simulink model "ARC_DTm"  (R2025b)
settings: Solver=FixedStepAuto  StartTime=0.0  StopTime=10080  FixedStep=1  RelTol=1e-3
PreLoadFcn:
  | %For Preload, set the working path
  | modelFolder = fileparts(which(bdroot));
  | addpath(genpath(modelFolder));
StartFcn:
  | tic
StopFcn:
  | fprintf("Sim Time: %.02f min", toc/60)
values from neighbouring files (symbols this model uses):
  batteryScenario = p.batteryScenario    [RUNSIM_ParameterSweep.m]    (also in _RUNSIM_ParameterSweep.m)
  Electricity_SalePriceModifier = 50/100    (= 0.5)    [RUNSIM_ParameterSweep.m]    (also in _RUNSIM_ParameterSweep.m)
  LUT = LUT_load.gamLUT    [RUNSIM_ParameterSweep.m]    (also in _RUNSIM_ParameterSweep.m)
  minimum_UF_system_flow = 5833    [RUNSIM_ParameterSweep.m]    (also in _RUNSIM_ParameterSweep.m)
  PROS1_recoveryrate = 61    [RUNSIM_ParameterSweep.m]    (also in _RUNSIM_ParameterSweep.m)
  PROS2_recoveryrate = 62    [RUNSIM_ParameterSweep.m]    (also in _RUNSIM_ParameterSweep.m)
  ROstabilization_time = p.ROstabilization_time    [RUNSIM_ParameterSweep.m]    (also in _RUNSIM_ParameterSweep.m)
  solarModifier = maximum_solar_generation / 300    [RUNSIM_ParameterSweep.m]    (also in _RUNSIM_ParameterSweep.m)
  TSRO_recoveryrate = 51    [RUNSIM_ParameterSweep.m]    (also in _RUNSIM_ParameterSweep.m)
  UF_RecoveryRate = 96    [RUNSIM_ParameterSweep.m]    (also in _RUNSIM_ParameterSweep.m)
undefined symbols (not defined in the file or in its folder): A_PROS1, A_PROS2, A_TSRO, B_PROS1, B_PROS2, B_TSRO, BW_Max_Time, BW_Max_Vol_gal, CEB_Max_Time, CEB_Max_Vol_gal, CIP_Max_Time, E, FF, h, L, w
libraries: simulink x40
(part 1 of 11)
settings Model: Creator=joshl  LastModifiedBy=joshl
settings DebuggingCC: AlgebraicLoopMsg=none  IntegerOverflowMsg=none
settings RTWCC: GenCodeOnly=on

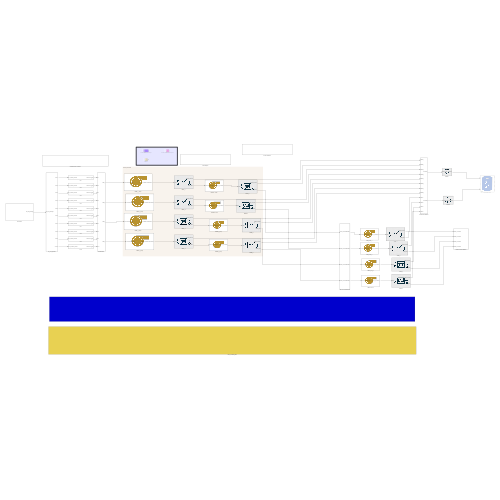
[thumbnail: Simulink's stored preview of the top-level diagram]
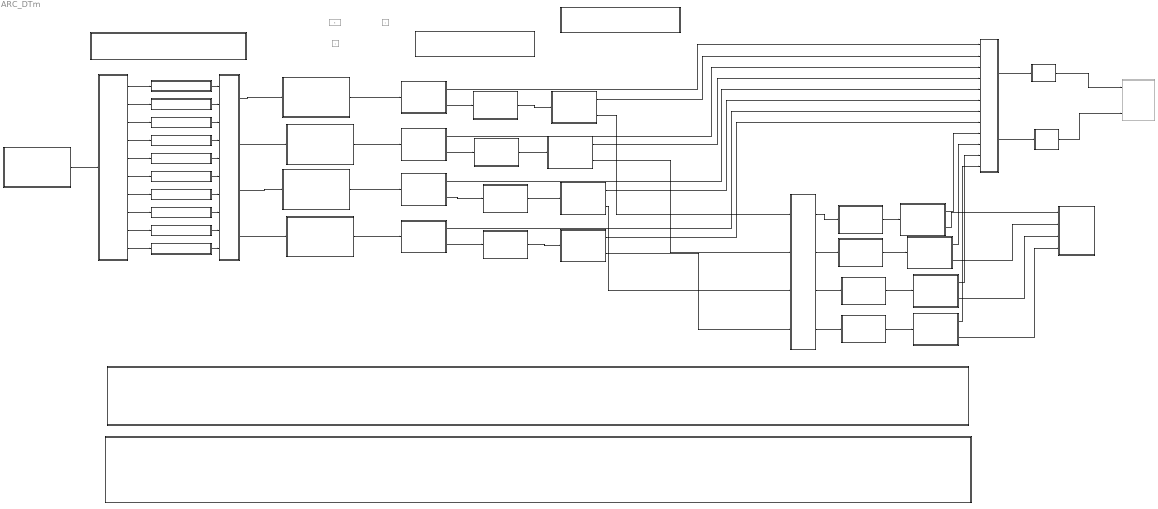
== system ARC_DTm ==
  note: Primary RO Skids
  note: LEGEND
  Constant Value from Analysis : Constant  Commented=on  Value=E
  Constant Value from Plant Specs : Constant  Commented=on
  PRO Concentrate Manifold : Subsystem
  PRO Manifolds : Subsystem
  PROS1_1 : Subsystem
      mask Display: image('ROmodule.png');
  PROS1_1_Pump : Subsystem
      mask Display: image('HydraulicPump.png');
  PROS1_2 : Subsystem
      mask Display: image('ROmodule.png');
  PROS1_2_Pump : Subsystem
      mask Display: image('HydraulicPump.png');
  PROS1_3 : Subsystem
      mask Display: image('ROmodule.png');
  PROS1_3_Pump : Subsystem
      mask Display: image('HydraulicPump.png');
  PROS1_4 : Subsystem
      mask Display: image('ROmodule.png');
  PROS1_4_Pump : Subsystem
      mask Display: image('HydraulicPump.png');
  PROS2_1 : Subsystem
      mask Display: image('ROmodule.png');
  PROS2_1_Pump : Subsystem
      mask Display: image('HydraulicPump.png');
  PROS2_2 : Subsystem
      mask Display: image('ROmodule.png');
  PROS2_2_Pump : Subsystem
      mask Display: image('HydraulicPump.png');
  PROS2_3 : Subsystem
      mask Display: image('ROmodule.png');
  PROS2_3_Pump : Subsystem
      mask Display: image('HydraulicPump.png');
  PROS2_4 : Subsystem
      mask Display: image('ROmodule.png');
  PROS2_4_Pump : Subsystem
      mask Display: image('HydraulicPump.png');
  Plant Setpoints : Subsystem
  Plant_LocalLoad_FMU : Subsystem
  Process Constants : Subsystem
  Product Water Tank : Subsystem  Commented=on  mask{lid=Closed, area=100, vol=500, volMax=0.750, volMin=.25, initVol=0.720, initTSS=43.0, InitSal=24.500, initT=31.500}
      mask prompts: lid "Open or Closed Lid?"; area "Surface Area of Tank (ft^2)"; vol "Volume of Tank (gal)"; volMax "Operational Max Volume (%)"; volMin "Operational Min Volume (%)"; initVol "Initial Storage Volume (%)"; initTSS "Initial TSS (ppm)"; InitSal "Initial Salinity (ppm)"; initT "Initial Temperature (*C)"
      mask TypeOptions lid: Open | Closed
      mask DialogControl Control1 Prompt: Raw Water Tank geometry definition
      mask Display: image('C:\Users\joshl\OneDrive - Colostate\Research\NAWI\Simulink Model\Icons\RawWaterTank.png'); % Use "Edit Image" on toolstrip to change.
  RO Permeate Manifold : Subsystem
  Setpoint : Constant  Commented=on
  Subsystem1 : Subsystem
  TSRO Concentrate Manifold : Subsystem
  TSRO_1 : Subsystem
      mask Display: image('ROmodule.png');
  TSRO_2 : Subsystem
      mask Display: image('ROmodule.png');
  TSRO_3 : Subsystem
      mask Display: image('ROmodule.png');
  TSRO_4 : Subsystem
      mask Display: image('ROmodule.png');
  TSRO_Pump_1 : Subsystem
      mask Display: image('HydraulicPump.png');
  TSRO_Pump_2 : Subsystem
      mask Display: image('HydraulicPump.png');
  TSRO_Pump_3 : Subsystem
      mask Display: image('HydraulicPump.png');
  TSRO_Pump_4 : Subsystem
      mask Display: image('HydraulicPump.png');
  UF Maintenance Coordinator : Subsystem
  UF Pumping : Subsystem
  UF1 : Subsystem
  UF10 : Subsystem
  UF2 : Subsystem
  UF3 : Subsystem
  UF4 : Subsystem
  UF5 : Subsystem
  UF6 : Subsystem
  UF7 : Subsystem
  UF8 : Subsystem
  UF9 : Subsystem
  UF_Feed_Manifold : Subsystem
  UVAOP 1 : Subsystem
      mask Display: image('11bcd1e1-7ab0-44c4-a430-d02249a16220.png');
  UVAOP 2 : Subsystem
      mask Display: image('11bcd1e1-7ab0-44c4-a430-d02249a16220.png');
  wires:
  PROS1_1_Pump/1(PRO1-1 FeedWater Characteristics) -> PROS1_1/1(Inflow)
  TSRO_1/1(TSRO_Permeate) -> RO Permeate Manifold/9(TSRO 1)
  UF Pumping/1(UF_Pump_Discharge) -> UF_Feed_Manifold/1(UF_Pump_Discharge)
  RO Permeate Manifold/1(To UVAOP1) -> UVAOP 1/1(feedFlow_gpm)
  RO Permeate Manifold/2(To UVAOP2) -> UVAOP 2/1(feedFlow_gpm)
  UVAOP 1/1(powerKW) -> Product Water Tank/1(Raw Water Inflow)
  UVAOP 2/1(powerKW) -> Product Water Tank/3(Pump Flow)
  PRO Manifolds/1(PRO_1) -> PROS1_1_Pump/1(S1 Feed Flow Rate (gpm))
  PROS1_1/1(PROS1_Permeate) -> RO Permeate Manifold/1(PROS1_1)
  PROS1_1/2(PROS1_Brine) -> PROS2_1_Pump/1(S2 Feed Flow Rate (gpm))
  PROS2_1/2(PROS2_Brine) -> PRO Concentrate Manifold/1(PRO1_Concentrate)
  PROS2_1/1(PROS2_Permeate) -> RO Permeate Manifold/2(PROS2_1)
  PRO Manifolds/2(PRO_2) -> PROS1_2_Pump/1(S1 Feed Flow Rate (gpm))
  PROS2_2/1(PROS2_Permeate) -> RO Permeate Manifold/4(PROS2_2)
  PROS2_2/2(PROS2_Brine) -> PRO Concentrate Manifold/2(PRO2_Concentrate)
  PRO Manifolds/3(PRO_3) -> PROS1_3_Pump/1(S1 Feed Flow Rate (gpm))
  PROS2_3/1(PROS2_Permeate) -> RO Permeate Manifold/6(PROS2_3)
  PROS2_3/2(PROS2_Brine) -> PRO Concentrate Manifold/3(PRO3_Concentrate)
  PROS2_4/1(PROS2_Permeate) -> RO Permeate Manifold/8(PROS2_4)
  PRO Manifolds/4(PRO_4) -> PROS1_4_Pump/1(S1 Feed Flow Rate (gpm))
  PROS2_4/2(PROS2_Brine) -> PRO Concentrate Manifold/4(PRO4_Concentrate)
  TSRO_Pump_1/1(TSRO_1_Feedwater) -> TSRO_1/1(Inflow)
  PRO Concentrate Manifold/1(To TSRO1) -> TSRO_Pump_1/1(S2 Feed Flow Rate (gpm))
  TSRO_1/2(TSRO_Brine) -> TSRO Concentrate Manifold/1(TSRO1_Concentrate)
  PROS2_1_Pump/1(PROS2_1_Feedwater) -> PROS2_1/1(Inflow)
  PROS1_2_Pump/1(PRO1-1 FeedWater Characteristics) -> PROS1_2/1(Inflow)
  PROS2_2_Pump/1(PROS2_2_Feedwater) -> PROS2_2/1(Inflow)
  PROS1_2/2(PROS1_Brine) -> PROS2_2_Pump/1(S2 Feed Flow Rate (gpm))
  PROS1_4_Pump/1(PRO1-1 FeedWater Characteristics) -> PROS1_4/1(Inflow)
  PROS2_4_Pump/1(PROS2_4_Feedwater) -> PROS2_4/1(Inflow)
  PROS1_4/2(PROS1_Brine) -> PROS2_4_Pump/1(S2 Feed Flow Rate (gpm))
  PROS1_2/1(PROS1_Permeate) -> RO Permeate Manifold/3(PROS1_2)
  PROS1_4/1(PROS1_Permeate) -> RO Permeate Manifold/7(PROS1_4)
  TSRO_Pump_2/1(TSRO_2_Feedwater) -> TSRO_2/1(Inflow)
  PRO Concentrate Manifold/2(To TSRO2) -> TSRO_Pump_2/1(S2 Feed Flow Rate (gpm))
  TSRO_2/1(TSRO_Permeate) -> RO Permeate Manifold/10(TSRO 2)
  TSRO_2/2(TSRO_Brine) -> TSRO Concentrate Manifold/2(TSRO2_Concentrate)
  TSRO_Pump_3/1(TSRO_3_Feedwater) -> TSRO_3/1(Inflow)
  PRO Concentrate Manifold/3(To TSRO3) -> TSRO_Pump_3/1(S2 Feed Flow Rate (gpm))
  TSRO_Pump_4/1(TSRO_4_Feedwater) -> TSRO_4/1(Inflow)
  PRO Concentrate Manifold/4(To TSRO4) -> TSRO_Pump_4/1(S2 Feed Flow Rate (gpm))
  TSRO_3/1(TSRO_Permeate) -> RO Permeate Manifold/11(TSRO 3)
  TSRO_3/2(TSRO_Brine) -> TSRO Concentrate Manifold/3(TSRO3_Concentrate)
  TSRO_4/1(TSRO_Permeate) -> RO Permeate Manifold/12(TSRO 4)
  TSRO_4/2(TSRO_Brine) -> TSRO Concentrate Manifold/4(TSRO4_Concentrate)
  PROS1_3/1(PROS1_Permeate) -> RO Permeate Manifold/5(PROS1_3)
  PROS2_3_Pump/1(PROS2_3_Feedwater) -> PROS2_3/1(Inflow)
  PROS1_3_Pump/1(PRO1-1 FeedWater Characteristics) -> PROS1_3/1(Inflow)
  PROS1_3/2(PROS1_Brine) -> PROS2_3_Pump/1(S2 Feed Flow Rate (gpm))
  UF_Feed_Manifold/10(To UF10) -> UF10/1(UF10_FeedFlow_Pressure)
  UF_Feed_Manifold/9(To UF9) -> UF9/1(UF9_FeedFlow_Pressure)
  UF_Feed_Manifold/7(To UF7) -> UF7/1(UF7_FeedFlow_Pressure)
  UF_Feed_Manifold/6(To UF6) -> UF6/1(UF6_FeedFlow_Pressure)
  UF_Feed_Manifold/5(To UF5) -> UF5/1(UF5_FeedFlow_Pressure)
  UF_Feed_Manifold/8(To UF8) -> UF8/1(UF8_FeedFlow_Pressure)
  UF_Feed_Manifold/3(To UF3) -> UF3/1(UF3_FeedFlow_Pressure)
  UF_Feed_Manifold/1(To UF1) -> UF1/1(UF1_FeedFlow_Pressure)
  UF_Feed_Manifold/2(To UF2) -> UF2/1(UF2_FeedFlow_Pressure)
  UF_Feed_Manifold/4(To UF4) -> UF4/1(UF4_FeedFlow_Pressure)
  UF10/1(Filtrate Flow (gpm)) -> PRO Manifolds/10(UF10)
  UF1/1(Filtrate Flow (gpm)) -> PRO Manifolds/1(UF1)
  UF2/1(Filtrate Flow (gpm)) -> PRO Manifolds/2(UF2)
  UF3/1(Filtrate Flow (gpm)) -> PRO Manifolds/3(UF3)
  UF4/1(Filtrate Flow (gpm)) -> PRO Manifolds/4(UF4)
  UF5/1(Filtrate Flow (gpm)) -> PRO Manifolds/5(UF5)
  UF6/1(Filtrate Flow (gpm)) -> PRO Manifolds/6(UF6)
  UF7/1(Filtrate Flow (gpm)) -> PRO Manifolds/7(UF7)
  UF8/1(Filtrate Flow (gpm)) -> PRO Manifolds/8(UF8)
  UF9/1(Filtrate Flow (gpm)) -> PRO Manifolds/9(UF9)

== system ARC_DTm/PRO Concentrate Manifold ==
  PRO1_Concentrate : Inport
  PRO2_Concentrate : Inport  Port=2
  PRO3_Concentrate : Inport  Port=3
  PRO4_Concentrate : Inport  Port=4
  Bus Creator{,1..3} (4 alike) : BusCreator  Inputs=3
  Bus Selector : BusSelector  OutputSignals=PROS2_1_BrineFlow_gpm,PROS2_1_BrineConductivity_gL,PROS2_1_ConcentratePressure_psi
  Bus Selector1 : BusSelector  OutputSignals=PROS2_2_BrineFlow_gpm,PROS2_2_BrineConductivity_gL,PROS2_2_ConcentratePressure_psi
  Bus Selector2 : BusSelector  OutputSignals=PROS2_3_BrineFlow_gpm,PROS2_3_BrineConductivity_gL,PROS2_3_ConcentratePressure_psi
  Bus Selector3 : BusSelector  OutputSignals=PROS2_4_BrineFlow_gpm,PROS2_4_BrineConductivity_gL,PROS2_4_ConcentratePressure_psi
  Constant : Constant  Value=0
  Constant1 : Constant  Value=ROstabilization_time
  Demux : Demux
  Divide : Product  Inputs=/*
  Divide1 : Product  Inputs=/*
  Max1 : MinMax  Function=max  Inputs=2
  Minus : Sum  Inputs=+-
  Number TSRO Units : MATLAB Function  TreatAsAtomicUnit=on
  PRO1_LoadingRate : Product
  PRO1_WeightedPressure : Product
  PRO2_LoadingRate : Product
  PRO2_WeightedPressure : Product
  PRO3_LoadingRate : Product
  PRO3_WeightedPressure : Product
  PRO4_LoadingRate : Product
  PRO4_WeightedPressure : Product
  PRO_TotalConcFlow_gpm : Sum  Inputs=++++
  PRO_TotalConcLoading : Sum  Inputs=++++
  PRO_WeightedConcPressure : Sum  Inputs=++++
  Scope : Scope  NumInputPorts=2
      settings: ActiveDisplayYMinimum=-1  ActiveDisplayYMaximum=1  DataLoggingVariableName=ScopeData19
  Scope1 : Scope
      settings: DataLoggingVariableName=ScopeData11
  Switch : Switch  Criteria=u2 > Threshold  SaturateOnIntegerOverflow=off  InputSameDT=off
  TSRO Feed Maximum (gpm) : Constant  Value=555
  TSRO_FeedWater : Scope  NumInputPorts=3
      settings: ActiveDisplayYMinimum=-14.033054409776806  ActiveDisplayYMaximum=126.29748968799129  DataLoggingVariableName=ScopeData42
  Unit Delay1 : UnitDelay  SampleTime=-1  HasFrameUpgradeWarning=on
  To TSRO1 : Outport
  To TSRO2 : Outport  Port=2
  To TSRO3 : Outport  Port=3
  To TSRO4 : Outport  Port=4
  tag scope: TSRO_UnitFlows=global
  wires:
  PRO3_Concentrate/1 -> Bus Selector2/1
  PRO1_Concentrate/1 -> Bus Selector/1
  PRO2_Concentrate/1 -> Bus Selector1/1
  PRO4_Concentrate/1 -> Bus Selector3/1
  PRO3_WeightedPressure/1 -> PRO_WeightedConcPressure/2
  Bus Selector/1 -> PRO_TotalConcFlow_gpm/1, PRO1_WeightedPressure/1, PRO1_LoadingRate/1  "<PROS2_1_BrineFlow_gpm>"
  Bus Selector/2 -> PRO1_LoadingRate/2  "<PROS2_1_BrineConductivity_gL>"
  Bus Selector2/1 -> PRO3_LoadingRate/1, PRO_TotalConcFlow_gpm/2, PRO3_WeightedPressure/1  "<PROS2_3_BrineFlow_gpm>"
  Bus Selector/3 -> PRO1_WeightedPressure/2  "<PROS2_1_ConcentratePressure_psi>"
  Bus Selector2/2 -> PRO3_LoadingRate/2  "<PROS2_3_BrineConductivity_gL>"
  PRO1_LoadingRate/1 -> PRO_TotalConcLoading/1
  Bus Selector2/3 -> PRO3_WeightedPressure/2  "<PROS2_3_ConcentratePressure_psi>"
  Bus Creator/1 -> To TSRO1/1
  Bus Selector3/1 -> PRO4_WeightedPressure/1, PRO_TotalConcFlow_gpm/3, PRO4_LoadingRate/1  "<PROS2_4_BrineFlow_gpm>"
  PRO1_WeightedPressure/1 -> PRO_WeightedConcPressure/1
  Bus Selector3/2 -> PRO4_LoadingRate/2  "<PROS2_4_BrineConductivity_gL>"
  Bus Selector3/3 -> PRO4_WeightedPressure/2  "<PROS2_4_ConcentratePressure_psi>"
  Bus Selector1/1 -> PRO2_LoadingRate/1, PRO_TotalConcFlow_gpm/4, PRO2_WeightedPressure/1  "<PROS2_2_BrineFlow_gpm>"
  Bus Selector1/2 -> PRO2_LoadingRate/2  "<PROS2_2_BrineConductivity_gL>"
  Bus Selector1/3 -> PRO2_WeightedPressure/2  "<PROS2_2_ConcentratePressure_psi>"
  PRO3_LoadingRate/1 -> PRO_TotalConcLoading/2
  PRO4_LoadingRate/1 -> PRO_TotalConcLoading/3
  Bus Creator1/1 -> To TSRO2/1
  Demux/1 -> Bus Creator/1  "TSRO_1_FeedFlow_gpm"
  PRO2_LoadingRate/1 -> PRO_TotalConcLoading/4
  PRO4_WeightedPressure/1 -> PRO_WeightedConcPressure/3
  PRO2_WeightedPressure/1 -> PRO_WeightedConcPressure/4
  TSRO Feed Maximum (gpm)/1 -> Number TSRO Units/1(max_flow_per_unit)
  PRO_TotalConcLoading/1 -> Divide/2
  PRO_TotalConcFlow_gpm/1 -> Number TSRO Units/2(flow_actual), Switch/2, Divide1/1, Divide/1
  PRO_WeightedConcPressure/1 -> Divide1/2
  Divide/1 -> Switch/1  "TSRO_FeedTDS_gL"
  Divide1/1 -> Minus/1  "TSRO_SuctionPressure_psi"
  Constant/1 -> Switch/3, Max1/2
  Switch/1 -> TSRO_FeedWater/2, Bus Creator3/2, Bus Creator2/2, Bus Creator/2, Bus Creator1/2  "TSRO_FeedTDS_gL"
  Demux/3 -> Bus Creator2/1  "TSRO_3_FeedFlow_gpm"
  Max1/1 -> Scope/1, Bus Creator/3, Bus Creator1/3, Bus Creator2/3, Bus Creator3/3, TSRO_FeedWater/1  "TSRO_SuctionPressure_psi"
  Demux/2 -> Bus Creator1/1  "TSRO_2_FeedFlow_gpm"
  Demux/4 -> Bus Creator3/1  "TSRO_4_FeedFlow_gpm"
  Bus Creator2/1 -> To TSRO3/1
  Bus Creator3/1 -> To TSRO4/1
  Unit Delay1/1 -> Number TSRO Units/4(prev_flows)
  Number TSRO Units/1(flows) -> Scope1/1, [TSRO_UnitFlows], Unit Delay1/1, TSRO_FeedWater/3, Demux/1  "TSRO_FeedFlows"
  [TSRO_Flow_SP] -> Number TSRO Units/3(flow_setpoint)
  Constant1/1 -> Number TSRO Units/6(ROstabilization_time)
  [Plant_StabilizationTime] -> Number TSRO Units/5(Stabilization_Time)
  [TSRO_Suction_PressureDrop_psi] -> Minus/2
  Minus/1 -> Max1/1

== system ARC_DTm/PRO Manifolds ==
  note: Pout = ( $\sum(Q_i * P_i)\\\sum(Q_i) - P_L$
  UF1 : Inport
  UF2 : Inport  Port=2
  UF3 : Inport  Port=3
  UF4 : Inport  Port=4
  UF5 : Inport  Port=5
  UF6 : Inport  Port=6
  UF7 : Inport  Port=7
  UF8 : Inport  Port=8
  UF9 : Inport  Port=9
  UF10 : Inport  Port=10
  Bus Creator{,1..3} (4 alike) : BusCreator  Inputs=2
  Demux : Demux
  Display : Display
  ROSuctionPressure : Constant  Value=35
  Sum : Sum  Inputs=+++++++++++
  PRO_1 : Outport
  PRO_2 : Outport  Port=2
  PRO_3 : Outport  Port=3
  PRO_4 : Outport  Port=4
  wires:
  Bus Creator/1 -> PRO_1/1
  ROSuctionPressure/1 -> Bus Creator2/2, Bus Creator3/2, Bus Creator1/2, Bus Creator/2  "PRO_SuctionPressure_psi"
  [PRO_FlowperUnit_gpm] -> Display/1, Demux/1  "PRO_FeedFlowRate_Vector"
  Demux/1 -> Bus Creator/1  "PROS1_1_FeedFlowRate_gpm"
  Bus Creator3/1 -> PRO_4/1
  Bus Creator2/1 -> PRO_3/1
  Demux/2 -> Bus Creator1/1  "PROS1_2_FeedFlowRate_gpm"
  Demux/3 -> Bus Creator2/1  "PROS1_3_FeedFlowRate_gpm"
  Demux/4 -> Bus Creator3/1  "PROS1_4_FeedFlowRate_gpm"
  Bus Creator1/1 -> PRO_2/1

== system ARC_DTm/PROS1_1 ==
  note: Units needed:
      | u = cm/sec
      | dh = cm
      | Concentrations = g/L
      | Jw_prev = L/m2/min
      |  = Q (Lpm) / Atot(m2)
      | T = oC
      | q = cm/sec =
      | Q (m3/sec) / Atot (m2)
  Inflow : Inport
  Brine Flow (gpm) : Sum  Inputs=-+
  Bus Creator : BusCreator  Inputs=2
  Bus Creator1 : BusCreator  Inputs=3
  Bus Selector : BusSelector  OutputSignals=S1 Feed Pressure (bar),PROS1_1_FeedFlowRate_gpm,S1 Feed Salinity (g/L),Feed Temperature (oC)
  Bus Selector1 : BusSelector  OutputSignals=PROS1_A,PROS1_B,PROS1_Area_m2
  Channel Area (m2) : Product  Inputs=4
  Elements per Vessel : Constant  Value=7
  Feed Channel Height (m) : Constant  Value=L
  Fouling Factor : Constant  Value=1-FF
  Gain : Gain  Gain=3.785
  Initial units : Gain  Gain=10^-8
  Jw_Previous : Memory  InitialCondition=.2949
  "L -> gal" : Gain  Gain=1/3.785
  L>m3 : Gain  Gain=1/1000
  MATLAB Function1 : MATLAB Function  TreatAsAtomicUnit=on
  MATLAB Function2 : MATLAB Function  TreatAsAtomicUnit=on
  Membrane Width (m) : Constant  Value=w
  Min : MinMax  Inputs=2
  Minus : Sum  Inputs=+-|
  Number of Vessels : Constant  Value=40
  Pa > Bar : Gain  Gain=100000
  Permeate Flow (gpm) : Product
  Product : Product  Inputs=*/
  Product2 : Product
  Q (L/min) : Gain  Gain=3.785
  Spacer Thickness (mm) : Constant  Value=h
  Subsystem : Subsystem
  bar>psi : Gain  Gain=1/.069
  cperm_previous : Memory  InitialCondition=.008
  gpm > L : Gain  Gain=3.785
  initial Units : Gain  Gain=10^-11
  m/min > cm/sec : Gain  Gain=100/60
  m3 > L : Gain  Gain=1000
  m3 > L1 : Gain  Gain=1000
  m>cm : Gain  Gain=100
  m>mm : Gain  Gain=1000
  mm>  cm : Gain  Gain=.1
  mm>m : Gain  Gain=.001
  psi to Bar : Gain  Gain=.069
  s > min : Gain  Gain=60
  s > min1 : Gain  Gain=60
  PROS1_Permeate : Outport
  PROS1_Brine : Outport  Port=2
  tag scope: PROS1_1_deltaPi=global
  wires:
  Number of Vessels/1 -> Channel Area (m2)/3
  [PROS1_MembraneConstants] -> Bus Selector1/1
  Minus/1 -> Bus Creator1/3  "PROS1_1_ConcentratePressure_psi"
  bar>psi/1 -> Minus/1  "PROS1_1_ConcentratePressure_psi"
  Membrane Width (m)/1 -> Channel Area (m2)/1, m>mm/1
  [RO_PermeatePressure] -> psi to Bar/1  "Permeate Pressure (psi)"
  Spacer Thickness (mm)/1 -> MATLAB Function1/2(h), mm>m/1
  Bus Selector1/3 -> Permeate Flow (gpm)/2  "<PROS1_Area_m2>"
  Inflow/1 -> Bus Selector/1
  Bus Selector1/1 -> initial Units/1  "<PROS1_A>"
  Bus Selector1/2 -> Initial units/1  "<PROS1_B>"
  initial Units/1 -> m3 > L/1
  psi to Bar/1 -> Min/2  "Pressure (bar)"
  Bus Selector/1 -> Min/1, Subsystem/2(<S1 Feed Pressure (bar)>), bar>psi/1  "<S1 Feed Pressure (bar)>"
  Bus Selector/2 -> Brine Flow (gpm)/2, Q (L/min)/1  "<PROS1_1_FeedFlowRate_gpm>"
  Subsystem/2(Permeate Salinity g/L) -> cperm_previous/1, Bus Creator/2, MATLAB Function2/1(cperm)  "PROS1_1_PermeateSalinity_gL"
  Bus Selector/3 -> MATLAB Function2/5(cfeed), Subsystem/6(<S1 Feed Salinity (g/L)>)  "<S1 Feed Salinity (g/L)>"
  Bus Selector/4 -> Subsystem/1(<Feed Temperature (oC)>)  "<Feed Temperature (oC)>"
  m/min > cm/sec/1 -> Subsystem/11(u)
  Initial units/1 -> m3 > L1/1
  Fouling Factor/1 -> Product2/2
  mm>m/1 -> Channel Area (m2)/2
  Min/1 -> Subsystem/3(Pperm)
  Pa > Bar/1 -> Product2/1  "Water Perm (L/m2/min/Bar)"
  m3 > L/1 -> s > min/1
  Q (L/min)/1 -> L>m3/1, MATLAB Function2/4(Qfeed)  "Qtot (L/min)"
  "L -> gal"/1 -> Permeate Flow (gpm)/1
  m3 > L1/1 -> s > min1/1
  Elements per Vessel/1 -> Channel Area (m2)/4
  [PROS2_Suction_PressureDrop_psi] -> Minus/2
  s > min/1 -> Pa > Bar/1
  s > min1/1 -> Subsystem/5(Salt Perm (L/m2/min))  "Salt Perm (L/m2/min)"
  m>mm/1 -> MATLAB Function1/1(W)
  MATLAB Function2/1(cbrine) -> Bus Creator1/2  "PROS1_1_BrineConductivity_gL"
  L>m3/1 -> Product/1
  Channel Area (m2)/1 -> Product/2
  cperm_previous/1 -> Subsystem/7(cperm)  "cperm"
  MATLAB Function1/1(dh) -> mm>  cm/1
  Feed Channel Height (m)/1 -> m>cm/1
  Product/1 -> m/min > cm/sec/1
  mm>  cm/1 -> Subsystem/9(dh)
  Product2/1 -> Subsystem/4(Water Perm (L/m2/min/Bar))  "Water Perm (L/m2/min/Bar)"
  m>cm/1 -> Subsystem/10(L)
  Subsystem/1(Permeate Flux Rate (L/min/m2)) -> Jw_Previous/1, "L -> gal"/1  "Permeate Flux Rate* (L/min.m2)"
  Subsystem/3(deltaPi_bar) -> [PROS1_1_deltaPi]
  gpm > L/1 -> MATLAB Function2/3(Qbrine)
  Jw_Previous/1 -> Subsystem/8(Jw)  "Jw"
  Gain/1 -> MATLAB Function2/2(Qperm)  "Predicted Permeate Flow (L/min)"
  Permeate Flow (gpm)/1 -> Bus Creator/1, Brine Flow (gpm)/1, Gain/1  "PROS1_1_PermeateFlow_gpm"
  Bus Creator/1 -> PROS1_Permeate/1  "PRO1_PermeateFlow"
  Brine Flow (gpm)/1 -> Bus Creator1/1, gpm > L/1  "PROS1_1_BrineFlow_gpm"
  Bus Creator1/1 -> PROS1_Brine/1  "PROS2_Feedwater"

== system ARC_DTm/PROS1_1_Pump ==
  note: Determine Needed Added Pressure
  note: gpm / (gpm/psi*ft2) / ft2
  S1 Feed Flow Rate (gpm) : Inport
  Bar > psi : Gain  Gain=1/.069
  Bus Creator : BusCreator  Inputs=4
  Bus Selector : BusSelector  OutputSignals=PROS1_A,PROS1_Area_m2
  Bus Selector1 : BusSelector  OutputSignals=PROS1_1_FeedFlowRate_gpm,PRO_SuctionPressure_psi
  Compare To Constant : simulink/Logic and Bit Operations/Compare To Constant  relop=>  const=1  OutDataTypeStr=boolean
  Constant : Constant  Value=0
  Display{,1..3} (4 alike) : Display
  Gain : Gain  Gain=.01
  Gain3 : Gain  Gain=10.76
  MATLAB Function : MATLAB Function  TreatAsAtomicUnit=on
  Memory : Memory
  PROS1_1_recoveryrate_per : Constant  Value=62
  Pa > psi : Gain  Gain=6895
  Product : Product  Inputs=**/
  Product1 : Product
  Product2 : Product
  Product3 : Product
  Scope : Scope  NumInputPorts=2
      settings: ActiveDisplayYMinimum=-21.182201274193289  ActiveDisplayYMaximum=190.63981146773963  DataLoggingVariableName=ScopeData13
  Scope1 : Scope  NumInputPorts=2
      settings: ActiveDisplayYMinimum=-1  ActiveDisplayYMaximum=1  DataLoggingVariableName=ScopeData14
  Scope3 : Scope
      settings: ActiveDisplayYMinimum=-1  ActiveDisplayYMaximum=1  DataLoggingVariableName=ScopeData16
  Sum : Sum  Inputs=|-+
  Sum1 : Sum  Inputs=|++
  Sum2 : Sum  Inputs=|++
  Switch : Switch  Criteria=u2 > Threshold  SaturateOnIntegerOverflow=off  InputSameDT=off
  m2 > ft2 : Gain  Gain=1/10.76
  m3 > gal : Gain  Gain=264.2
  m3/m2/s/Pa : Gain  Gain=10^-11
  psi to Bar : Gain  Gain=.069
  psi>ft : Gain  Gain=2.31
  s > min : Gain  Gain=60
  PRO1-1 FeedWater Characteristics : Outport
  tag scope: PROS1_1_Power_kW=global
  wires:
  Bus Selector1/2 -> Sum/1  "<PRO_SuctionPressure_psi>"
  Product2/1 -> Bus Creator/1  "S1 Feed Salinity (g/L)"
  [T] -> Bus Creator/2  "Feed Temperature (oC)"
  psi to Bar/1 -> Product3/2  "S1 Feed Pressure (bar)"
  Bus Creator/1 -> PRO1-1 FeedWater Characteristics/1
  [PROS1_1_deltaPi] -> Bar > psi/1
  Switch/1 -> Sum1/2
  Sum1/1 -> Scope3/1, Sum2/1  "Net Opposing Pressure (psi)"
  Bar > psi/1 -> Memory/1
  [PROS1_MembraneConstants] -> Bus Selector/1
  Bus Selector/1 -> m3/m2/s/Pa/1  "<PROS1_A>"
  PROS1_1_recoveryrate_per/1 -> Gain/1
  Gain/1 -> Product/2
  Product/1 -> Sum2/2  "PROS1_1_RequiredNDP_psi"
  m3 > gal/1 -> s > min/1
  s > min/1 -> Pa > psi/1
  m3/m2/s/Pa/1 -> m3 > gal/1
  Pa > psi/1 -> m2 > ft2/1  "Water Perm (gpm/m2/bar)"
  m2 > ft2/1 -> Product1/1  "PROS1_WaterPermeability_gpm_psi_ft2"
  Sum2/1 -> psi to Bar/1, Sum/2, Scope1/1  "PROS1_1_FeedPressure_psi"
  Bus Selector/2 -> Gain3/1  "<PROS1_Area_m2>"
  Gain3/1 -> Display/1, Product1/2  "PROS1_Area_ft2"
  S1 Feed Flow Rate (gpm)/1 -> Bus Selector1/1  "InflowRate (gpm)"
  Sum/1 -> Scope1/2, psi>ft/1
  psi>ft/1 -> Display3/1, MATLAB Function/2(h_des)
  MATLAB Function/2(power) -> [PROS1_1_Power_kW], Scope/1  "PROS1_1_Power_kW"
  Memory/1 -> Sum1/1
  Product1/1 -> Product/3
  MATLAB Function/1(speed) -> Display2/1
  Bus Selector1/1 -> Display1/1, Scope/2, MATLAB Function/1(Q_des), Compare To Constant/1, Bus Creator/3, Switch/2, Product/1  "<PROS1_1_FeedFlowRate_gpm>"
  [PROS1_FeedTDS_gL] -> Product2/1  "S1 Feed Salinity (g/L)"
  Compare To Constant/1 -> Product3/1, Product2/2
  Product3/1 -> Bus Creator/4  "S1 Feed Pressure (bar)"
  [RO_PermeatePressure] -> Switch/1
  Constant/1 -> Switch/3

== system ARC_DTm/PROS1_2 ==
  note: Units needed:
      | u = cm/sec
      | dh = cm
      | Concentrations = g/L
      | Jw_prev = L/m2/min
      |  = Q (Lpm) / Atot(m2)
      | T = oC
      | q = cm/sec =
      | Q (m3/sec) / Atot (m2)
  Inflow : Inport
  Brine Flow (gpm) : Sum  Inputs=-+
  Bus Creator : BusCreator  Inputs=2
  Bus Creator1 : BusCreator  Inputs=3
  Bus Selector : BusSelector  OutputSignals=S1 Feed Pressure (bar),PROS1_2_FeedFlowRate_gpm,S1 Feed Salinity (g/L),Feed Temperature (oC)
  Bus Selector1 : BusSelector  OutputSignals=PROS1_A,PROS1_B,PROS1_Area_m2
  Channel Area (m2) : Product  Inputs=4
  Elements per Vessel : Constant  Value=7
  Feed Channel Height (m) : Constant  Value=L
  Fouling Factor : Constant  Value=1-FF
  Gain : Gain  Gain=3.785
  Initial units : Gain  Gain=10^-8
  Jw_Previous : Memory  InitialCondition=.2949
  "L -> gal" : Gain  Gain=1/3.785
  L>m3 : Gain  Gain=1/1000
  MATLAB Function1 : MATLAB Function  TreatAsAtomicUnit=on
  MATLAB Function2 : MATLAB Function  TreatAsAtomicUnit=on
  Membrane Width (m) : Constant  Value=w
  Min : MinMax  Inputs=2
  Minus : Sum  Inputs=+-|
  Number of Vessels : Constant  Value=40
  Pa > Bar : Gain  Gain=100000
  Permeate Flow (gpm) : Product
  Product : Product  Inputs=*/
  Product2 : Product
  Q (L/min) : Gain  Gain=3.785
  Spacer Thickness (mm) : Constant  Value=h
  Subsystem : Subsystem
  bar>psi : Gain  Gain=1/.069
  cperm_previous : Memory  InitialCondition=.008
  gpm > L : Gain  Gain=3.785
  initial Units : Gain  Gain=10^-11
  m/min > cm/sec : Gain  Gain=100/60
  m3 > L : Gain  Gain=1000
  m3 > L1 : Gain  Gain=1000
  m>cm : Gain  Gain=100
  m>mm : Gain  Gain=1000
  mm>  cm : Gain  Gain=.1
  mm>m : Gain  Gain=.001
  psi to Bar : Gain  Gain=.069
  s > min : Gain  Gain=60
  s > min1 : Gain  Gain=60
  PROS1_Permeate : Outport
  PROS1_Brine : Outport  Port=2
  tag scope: PROS1_2_deltaPi=global
  wires:
  Number of Vessels/1 -> Channel Area (m2)/3
  [PROS1_MembraneConstants] -> Bus Selector1/1
  Minus/1 -> Bus Creator1/3  "PROS1_2_ConcentratePressure_psi"
  bar>psi/1 -> Minus/1  "PROS1_2_ConcentratePressure_psi"
  Membrane Width (m)/1 -> Channel Area (m2)/1, m>mm/1
  [RO_PermeatePressure] -> psi to Bar/1  "Permeate Pressure (psi)"
  Spacer Thickness (mm)/1 -> mm>m/1, MATLAB Function1/2(h)
  Bus Selector1/3 -> Permeate Flow (gpm)/2  "<PROS1_Area_m2>"
  Inflow/1 -> Bus Selector/1
  Bus Selector1/1 -> initial Units/1  "<PROS1_A>"
  Bus Selector1/2 -> Initial units/1  "<PROS1_B>"
  initial Units/1 -> m3 > L/1
  psi to Bar/1 -> Min/2  "Pressure (bar)"
  Bus Selector/1 -> Min/1, Subsystem/2(<S1 Feed Pressure (bar)>), bar>psi/1  "<S1 Feed Pressure (bar)>"
  Bus Selector/2 -> Brine Flow (gpm)/2, Q (L/min)/1  "<PROS1_2_FeedFlowRate_gpm>"
  Subsystem/2(Permeate Salinity g/L) -> Bus Creator/2, MATLAB Function2/1(cperm), cperm_previous/1  "PROS1_2_PermeateSalinity_gL"
  Bus Selector/3 -> MATLAB Function2/5(cfeed), Subsystem/6(<S1 Feed Salinity (g/L)>)  "<S1 Feed Salinity (g/L)>"
  Bus Selector/4 -> Subsystem/1(<Feed Temperature (oC)>)  "<Feed Temperature (oC)>"
  m/min > cm/sec/1 -> Subsystem/11(u)
  Initial units/1 -> m3 > L1/1
  Fouling Factor/1 -> Product2/2
  mm>m/1 -> Channel Area (m2)/2
  Min/1 -> Subsystem/3(Pperm)
  Pa > Bar/1 -> Product2/1  "Water Perm (L/m2/min/Bar)"
  m3 > L/1 -> s > min/1
  Q (L/min)/1 -> L>m3/1, MATLAB Function2/4(Qfeed)  "Qtot (L/min)"
  "L -> gal"/1 -> Permeate Flow (gpm)/1
  m3 > L1/1 -> s > min1/1
  Elements per Vessel/1 -> Channel Area (m2)/4
  [PROS2_Suction_PressureDrop_psi] -> Minus/2
  s > min/1 -> Pa > Bar/1
  s > min1/1 -> Subsystem/5(Salt Perm (L/m2/min))  "Salt Perm (L/m2/min)"
  m>mm/1 -> MATLAB Function1/1(W)
  MATLAB Function2/1(cbrine) -> Bus Creator1/2  "PROS1_2_BrineConductivity_gL"
  L>m3/1 -> Product/1
  Channel Area (m2)/1 -> Product/2
  cperm_previous/1 -> Subsystem/7(cperm)  "cperm"
  MATLAB Function1/1(dh) -> mm>  cm/1
  Feed Channel Height (m)/1 -> m>cm/1
  Product/1 -> m/min > cm/sec/1
  mm>  cm/1 -> Subsystem/9(dh)
  Product2/1 -> Subsystem/4(Water Perm (L/m2/min/Bar))  "Water Perm (L/m2/min/Bar)"
  m>cm/1 -> Subsystem/10(L)
  Subsystem/1(Permeate Flux Rate (L/min/m2)) -> Jw_Previous/1, "L -> gal"/1  "Permeate Flux Rate* (L/min.m2)"
  Subsystem/3(deltaPi_bar) -> [PROS1_2_deltaPi]
  gpm > L/1 -> MATLAB Function2/3(Qbrine)
  Jw_Previous/1 -> Subsystem/8(Jw)  "Jw"
  Gain/1 -> MATLAB Function2/2(Qperm)  "Predicted Permeate Flow (L/min)"
  Permeate Flow (gpm)/1 -> Brine Flow (gpm)/1, Bus Creator/1, Gain/1  "PROS1_2_PermeateFlow_gpm"
  Bus Creator/1 -> PROS1_Permeate/1  "PRO1_PermeateFlow"
  Brine Flow (gpm)/1 -> Bus Creator1/1, gpm > L/1  "PROS1_2_BrineFlow_gpm"
  Bus Creator1/1 -> PROS1_Brine/1  "PROS1_Feedwater"

== system ARC_DTm/PROS1_2_Pump ==
  note: Determine Needed Added Pressure
  note: gpm / (gpm/psi*ft2) / ft2
  S1 Feed Flow Rate (gpm) : Inport
  Bar > psi : Gain  Gain=1/.069
  Bus Creator : BusCreator  Inputs=4
  Bus Selector : BusSelector  OutputSignals=PROS1_A,PROS1_Area_m2
  Bus Selector1 : BusSelector  OutputSignals=PROS1_2_FeedFlowRate_gpm,PRO_SuctionPressure_psi
  Compare To Constant : simulink/Logic and Bit Operations/Compare To Constant  relop=>  const=1  OutDataTypeStr=boolean
  Constant : Constant  Value=0
  Display{,1..3} (4 alike) : Display
  Gain : Gain  Gain=.01
  Gain3 : Gain  Gain=10.76
  MATLAB Function : MATLAB Function  TreatAsAtomicUnit=on
  Memory : Memory
  PROS1_2_recoveryrate_per : Constant  Value=62
  Pa > psi : Gain  Gain=6895
  Product : Product  Inputs=**/
  Product1 : Product
  Product2 : Product
  Product3 : Product
  Scope : Scope  NumInputPorts=2
      settings: ActiveDisplayYMinimum=-21.182201274193289  ActiveDisplayYMaximum=190.63981146773963  DataLoggingVariableName=ScopeData13
  Scope1 : Scope  NumInputPorts=2
      settings: ActiveDisplayYMinimum=-1  ActiveDisplayYMaximum=1  DataLoggingVariableName=ScopeData14
  Scope3 : Scope
      settings: ActiveDisplayYMinimum=-1  ActiveDisplayYMaximum=1  DataLoggingVariableName=ScopeData16
  Sum : Sum  Inputs=|-+
  Sum1 : Sum  Inputs=|++
  Sum2 : Sum  Inputs=|++
  Switch : Switch  Criteria=u2 > Threshold  SaturateOnIntegerOverflow=off  InputSameDT=off
  m2 > ft2 : Gain  Gain=1/10.76
  m3 > gal : Gain  Gain=264.2
  m3/m2/s/Pa : Gain  Gain=10^-11
  psi to Bar : Gain  Gain=.069
  psi>ft : Gain  Gain=2.31
  s > min : Gain  Gain=60
  PRO1-1 FeedWater Characteristics : Outport
  tag scope: PROS1_2_Power_kW=global
  wires:
  Bus Selector1/2 -> Sum/1  "<PRO_SuctionPressure_psi>"
  Product2/1 -> Bus Creator/1  "S1 Feed Salinity (g/L)"
  [T] -> Bus Creator/2  "Feed Temperature (oC)"
  psi to Bar/1 -> Product3/2  "S1 Feed Pressure (bar)"
  Bus Creator/1 -> PRO1-1 FeedWater Characteristics/1
  [PROS1_2_deltaPi] -> Bar > psi/1
  Switch/1 -> Sum1/2
  Sum1/1 -> Scope3/1, Sum2/1  "Net Opposing Pressure (psi)"
  Bar > psi/1 -> Memory/1
  [PROS1_MembraneConstants] -> Bus Selector/1
  Bus Selector/1 -> m3/m2/s/Pa/1  "<PROS1_A>"
  PROS1_2_recoveryrate_per/1 -> Gain/1
  Gain/1 -> Product/2
  Product/1 -> Sum2/2  "PROS1_2_RequiredNDP_psi"
  m3 > gal/1 -> s > min/1
  s > min/1 -> Pa > psi/1
  m3/m2/s/Pa/1 -> m3 > gal/1
  Pa > psi/1 -> m2 > ft2/1  "Water Perm (gpm/m2/bar)"
  m2 > ft2/1 -> Product1/1  "PROS1_WaterPermeability_gpm_psi_ft2"
  Sum2/1 -> psi to Bar/1, Sum/2, Scope1/1  "PROS1_2_FeedPressure_psi"
  Bus Selector/2 -> Gain3/1  "<PROS1_Area_m2>"
  Gain3/1 -> Display/1, Product1/2  "PROS1_Area_ft2"
  S1 Feed Flow Rate (gpm)/1 -> Bus Selector1/1  "InflowRate (gpm)"
  Sum/1 -> Scope1/2, psi>ft/1
  psi>ft/1 -> Display3/1, MATLAB Function/2(h_des)
  MATLAB Function/2(power) -> [PROS1_2_Power_kW], Scope/1  "PROS1_2_Power_kW"
  Memory/1 -> Sum1/1
  Product1/1 -> Product/3
  MATLAB Function/1(speed) -> Display2/1
  Bus Selector1/1 -> Display1/1, Scope/2, MATLAB Function/1(Q_des), Compare To Constant/1, Bus Creator/3, Switch/2, Product/1  "<PROS1_2_FeedFlowRate_gpm>"
  [PROS1_FeedTDS_gL] -> Product2/1  "S1 Feed Salinity (g/L)"
  Compare To Constant/1 -> Product3/1, Product2/2
  Product3/1 -> Bus Creator/4  "S1 Feed Pressure (bar)"
  [RO_PermeatePressure] -> Switch/1
  Constant/1 -> Switch/3

== system ARC_DTm/PROS1_3 ==
  note: Units needed:
      | u = cm/sec
      | dh = cm
      | Concentrations = g/L
      | Jw_prev = L/m2/min
      |  = Q (Lpm) / Atot(m2)
      | T = oC
      | q = cm/sec =
      | Q (m3/sec) / Atot (m2)
  Inflow : Inport
  Brine Flow (gpm) : Sum  Inputs=-+
  Bus Creator : BusCreator  Inputs=2
  Bus Creator1 : BusCreator  Inputs=3
  Bus Selector : BusSelector  OutputSignals=S1 Feed Pressure (bar),PROS1_3_FeedFlowRate_gpm,S1 Feed Salinity (g/L),Feed Temperature (oC)
  Bus Selector1 : BusSelector  OutputSignals=PROS1_A,PROS1_B,PROS1_Area_m2
  Channel Area (m2) : Product  Inputs=4
  Elements per Vessel : Constant  Value=7
  Feed Channel Height (m) : Constant  Value=L
  Fouling Factor : Constant  Value=1-FF
  Gain : Gain  Gain=3.785
  Initial units : Gain  Gain=10^-8
  Jw_Previous : Memory  InitialCondition=.2949
  "L -> gal" : Gain  Gain=1/3.785
  L>m3 : Gain  Gain=1/1000
  MATLAB Function1 : MATLAB Function  TreatAsAtomicUnit=on
  MATLAB Function2 : MATLAB Function  TreatAsAtomicUnit=on
  Membrane Width (m) : Constant  Value=w
  Min : MinMax  Inputs=2
  Minus : Sum  Inputs=+-|
  Number of Vessels : Constant  Value=40
  Pa > Bar : Gain  Gain=100000
  Permeate Flow (gpm) : Product
  Product : Product  Inputs=*/
  Product2 : Product
  Q (L/min) : Gain  Gain=3.785
  Scope1 : Scope  NumInputPorts=2
      settings: ActiveDisplayYMinimum=-1277.4374999999993  ActiveDisplayYMaximum=11496.937499999996  DataLoggingVariableName=ScopeData29
  Spacer Thickness (mm) : Constant  Value=h
  Subsystem : Subsystem
  bar>psi : Gain  Gain=1/.069
  cperm_previous : Memory  InitialCondition=.008
  gpm > L : Gain  Gain=3.785
  initial Units : Gain  Gain=10^-11
  m/min > cm/sec : Gain  Gain=100/60
  m3 > L : Gain  Gain=1000
  m3 > L1 : Gain  Gain=1000
  m>cm : Gain  Gain=100
  m>mm : Gain  Gain=1000
  mm>  cm : Gain  Gain=.1
  mm>m : Gain  Gain=.001
  psi to Bar : Gain  Gain=.069
  s > min : Gain  Gain=60
  s > min1 : Gain  Gain=60
  PROS1_Permeate : Outport
  PROS1_Brine : Outport  Port=2
  tag scope: PROS1_3_deltaPi=global
  wires:
  Number of Vessels/1 -> Channel Area (m2)/3
  [PROS1_MembraneConstants] -> Bus Selector1/1
  Minus/1 -> Bus Creator1/3  "PROS1_3_ConcentratePressure_psi"
  bar>psi/1 -> Minus/1  "PROS1_3_ConcentratePressure_psi"
  Membrane Width (m)/1 -> Channel Area (m2)/1, m>mm/1
  [RO_PermeatePressure] -> psi to Bar/1  "Permeate Pressure (psi)"
  Spacer Thickness (mm)/1 -> MATLAB Function1/2(h), mm>m/1
  Bus Selector1/3 -> Permeate Flow (gpm)/2  "<PROS1_Area_m2>"
  Inflow/1 -> Bus Selector/1
  Bus Selector1/1 -> initial Units/1  "<PROS1_A>"
  Bus Selector1/2 -> Initial units/1  "<PROS1_B>"
  initial Units/1 -> m3 > L/1
  psi to Bar/1 -> Min/2  "Pressure (bar)"
  Bus Selector/1 -> Min/1, Subsystem/2(<S1 Feed Pressure (bar)>), bar>psi/1  "<S1 Feed Pressure (bar)>"
  Bus Selector/2 -> Brine Flow (gpm)/2, Q (L/min)/1  "<PROS1_3_FeedFlowRate_gpm>"
  Subsystem/2(Permeate Salinity g/L) -> cperm_previous/1, Bus Creator/2, MATLAB Function2/1(cperm)  "PROS1_3_PermeateSalinity_gL"
  Bus Selector/3 -> MATLAB Function2/5(cfeed), Scope1/2, Subsystem/6(<S1 Feed Salinity (g/L)>)  "<S1 Feed Salinity (g/L)>"
  Bus Selector/4 -> Subsystem/1(<Feed Temperature (oC)>)  "<Feed Temperature (oC)>"
  m/min > cm/sec/1 -> Subsystem/11(u)
  Initial units/1 -> m3 > L1/1
  Fouling Factor/1 -> Product2/2
  mm>m/1 -> Channel Area (m2)/2
  Min/1 -> Subsystem/3(Pperm)
  Pa > Bar/1 -> Product2/1  "Water Perm (L/m2/min/Bar)"
  m3 > L/1 -> s > min/1
  Q (L/min)/1 -> Scope1/1, L>m3/1, MATLAB Function2/4(Qfeed)  "Qtot (L/min)"
  "L -> gal"/1 -> Permeate Flow (gpm)/1
  m3 > L1/1 -> s > min1/1
  Elements per Vessel/1 -> Channel Area (m2)/4
  [PROS2_Suction_PressureDrop_psi] -> Minus/2
  s > min/1 -> Pa > Bar/1
  s > min1/1 -> Subsystem/5(Salt Perm (L/m2/min))  "Salt Perm (L/m2/min)"
  m>mm/1 -> MATLAB Function1/1(W)
  MATLAB Function2/1(cbrine) -> Bus Creator1/2  "PROS1_3_BrineConductivity_gL"
  L>m3/1 -> Product/1
  Channel Area (m2)/1 -> Product/2
  cperm_previous/1 -> Subsystem/7(cperm)  "cperm"
  MATLAB Function1/1(dh) -> mm>  cm/1
  Feed Channel Height (m)/1 -> m>cm/1
  Product/1 -> m/min > cm/sec/1
  mm>  cm/1 -> Subsystem/9(dh)
  Product2/1 -> Subsystem/4(Water Perm (L/m2/min/Bar))  "Water Perm (L/m2/min/Bar)"
  m>cm/1 -> Subsystem/10(L)
  Subsystem/1(Permeate Flux Rate (L/min/m2)) -> Jw_Previous/1, "L -> gal"/1  "Permeate Flux Rate* (L/min.m2)"
  Subsystem/3(deltaPi_bar) -> [PROS1_3_deltaPi]
  gpm > L/1 -> MATLAB Function2/3(Qbrine)
  Jw_Previous/1 -> Subsystem/8(Jw)  "Jw"
  Gain/1 -> MATLAB Function2/2(Qperm)  "Predicted Permeate Flow (L/min)"
  Permeate Flow (gpm)/1 -> Brine Flow (gpm)/1, Bus Creator/1, Gain/1  "PROS1_3_PermeateFlow_gpm"
  Bus Creator/1 -> PROS1_Permeate/1  "PRO1_PermeateFlow"
  Brine Flow (gpm)/1 -> Bus Creator1/1, gpm > L/1  "PROS1_3_BrineFlow_gpm"
  Bus Creator1/1 -> PROS1_Brine/1  "PROS1_Feedwater"

== system ARC_DTm/PROS1_3_Pump ==
  note: Determine Needed Added Pressure
  note: gpm / (gpm/psi*ft2) / ft2
  S1 Feed Flow Rate (gpm) : Inport
  Bar > psi : Gain  Gain=1/.069
  Bus Creator : BusCreator  Inputs=4
  Bus Selector : BusSelector  OutputSignals=PROS1_A,PROS1_Area_m2
  Bus Selector1 : BusSelector  OutputSignals=PROS1_3_FeedFlowRate_gpm,PRO_SuctionPressure_psi
  Compare To Constant : simulink/Logic and Bit Operations/Compare To Constant  relop=>  const=1  OutDataTypeStr=boolean
  Constant : Constant  Value=0
  Display{,1..3} (4 alike) : Display
  Gain : Gain  Gain=.01
  Gain3 : Gain  Gain=10.76
  MATLAB Function : MATLAB Function  TreatAsAtomicUnit=on
  Memory : Memory
  PROS1_3_recoveryrate_per : Constant  Value=62
  Pa > psi : Gain  Gain=6895
  Product : Product  Inputs=**/
  Product1 : Product
  Product2 : Product
  Product3 : Product
  Scope : Scope  NumInputPorts=2
      settings: ActiveDisplayYMinimum=-21.182201274193289  ActiveDisplayYMaximum=190.63981146773963  DataLoggingVariableName=ScopeData13
  Scope1 : Scope  NumInputPorts=2
      settings: ActiveDisplayYMinimum=-1  ActiveDisplayYMaximum=1  DataLoggingVariableName=ScopeData14
  Scope3 : Scope
      settings: ActiveDisplayYMinimum=-1  ActiveDisplayYMaximum=1  DataLoggingVariableName=ScopeData16
  Sum : Sum  Inputs=|-+
  Sum1 : Sum  Inputs=|++
  Sum2 : Sum  Inputs=|++
  Switch : Switch  Criteria=u2 > Threshold  SaturateOnIntegerOverflow=off  InputSameDT=off
  m2 > ft2 : Gain  Gain=1/10.76
  m3 > gal : Gain  Gain=264.2
  m3/m2/s/Pa : Gain  Gain=10^-11
  psi to Bar : Gain  Gain=.069
  psi>ft : Gain  Gain=2.31
  s > min : Gain  Gain=60
  PRO1-1 FeedWater Characteristics : Outport
  tag scope: PROS1_3_Power_kW=global
  wires:
  Bus Selector1/2 -> Sum/1  "<PRO_SuctionPressure_psi>"
  Product2/1 -> Bus Creator/1  "S1 Feed Salinity (g/L)"
  [T] -> Bus Creator/2  "Feed Temperature (oC)"
  psi to Bar/1 -> Product3/2  "S1 Feed Pressure (bar)"
  Bus Creator/1 -> PRO1-1 FeedWater Characteristics/1
  [PROS1_3_deltaPi] -> Bar > psi/1
  Switch/1 -> Sum1/2
  Sum1/1 -> Scope3/1, Sum2/1  "Net Opposing Pressure (psi)"
  Bar > psi/1 -> Memory/1
  [PROS1_MembraneConstants] -> Bus Selector/1
  Bus Selector/1 -> m3/m2/s/Pa/1  "<PROS1_A>"
  PROS1_3_recoveryrate_per/1 -> Gain/1
  Gain/1 -> Product/2
  Product/1 -> Sum2/2  "PROS1_3_RequiredNDP_psi"
  m3 > gal/1 -> s > min/1
  s > min/1 -> Pa > psi/1
  m3/m2/s/Pa/1 -> m3 > gal/1
  Pa > psi/1 -> m2 > ft2/1  "Water Perm (gpm/m2/bar)"
  m2 > ft2/1 -> Product1/1  "PROS1_WaterPermeability_gpm_psi_ft2"
  Sum2/1 -> psi to Bar/1, Sum/2, Scope1/1  "PROS1_3_FeedPressure_psi"
  Bus Selector/2 -> Gain3/1  "<PROS1_Area_m2>"
  Gain3/1 -> Display/1, Product1/2  "PROS1_Area_ft2"
  S1 Feed Flow Rate (gpm)/1 -> Bus Selector1/1  "InflowRate (gpm)"
  Sum/1 -> Scope1/2, psi>ft/1
  psi>ft/1 -> Display3/1, MATLAB Function/2(h_des)
  MATLAB Function/2(power) -> [PROS1_3_Power_kW], Scope/1  "PROS1_3_Power_kW"
  Memory/1 -> Sum1/1
  Product1/1 -> Product/3
  MATLAB Function/1(speed) -> Display2/1
  Bus Selector1/1 -> Display1/1, Scope/2, MATLAB Function/1(Q_des), Compare To Constant/1, Bus Creator/3, Switch/2, Product/1  "<PROS1_3_FeedFlowRate_gpm>"
  [PROS1_FeedTDS_gL] -> Product2/1  "S1 Feed Salinity (g/L)"
  Compare To Constant/1 -> Product3/1, Product2/2
  Product3/1 -> Bus Creator/4  "S1 Feed Pressure (bar)"
  [RO_PermeatePressure] -> Switch/1
  Constant/1 -> Switch/3

== system ARC_DTm/PROS1_4 ==
  note: Units needed:
      | u = cm/sec
      | dh = cm
      | Concentrations = g/L
      | Jw_prev = L/m2/min
      |  = Q (Lpm) / Atot(m2)
      | T = oC
      | q = cm/sec =
      | Q (m3/sec) / Atot (m2)
  Inflow : Inport
  Brine Flow (gpm) : Sum  Inputs=-+
  Bus Creator : BusCreator  Inputs=2
  Bus Creator1 : BusCreator  Inputs=3
  Bus Selector : BusSelector  OutputSignals=S1 Feed Pressure (bar),PROS1_4_FeedFlowRate_gpm,S1 Feed Salinity (g/L),Feed Temperature (oC)
  Bus Selector1 : BusSelector  OutputSignals=PROS1_A,PROS1_B,PROS1_Area_m2
  Channel Area (m2) : Product  Inputs=4
  Elements per Vessel : Constant  Value=7
  Feed Channel Height (m) : Constant  Value=L
  Fouling Factor : Constant  Value=1-FF
  Gain : Gain  Gain=3.785
  Initial units : Gain  Gain=10^-8
  Jw_Previous : Memory  InitialCondition=.2949
  "L -> gal" : Gain  Gain=1/3.785
  L>m3 : Gain  Gain=1/1000
  MATLAB Function1 : MATLAB Function  TreatAsAtomicUnit=on
  MATLAB Function2 : MATLAB Function  TreatAsAtomicUnit=on
  Membrane Width (m) : Constant  Value=w
  Min : MinMax  Inputs=2
  Minus : Sum  Inputs=+-|
  Number of Vessels : Constant  Value=40
  Pa > Bar : Gain  Gain=100000
  Permeate Flow (gpm) : Product
  Product : Product  Inputs=*/
  Product2 : Product
  Q (L/min) : Gain  Gain=3.785
  Scope1 : Scope  NumInputPorts=2
      settings: ActiveDisplayYMinimum=-1277.4374999999993  ActiveDisplayYMaximum=11496.937499999996  DataLoggingVariableName=ScopeData29
  Spacer Thickness (mm) : Constant  Value=h
  Subsystem : Subsystem
  bar>psi : Gain  Gain=1/.069
  cperm_previous : Memory  InitialCondition=.008
  gpm > L : Gain  Gain=3.785
  initial Units : Gain  Gain=10^-11
  m/min > cm/sec : Gain  Gain=100/60
  m3 > L : Gain  Gain=1000
  m3 > L1 : Gain  Gain=1000
  m>cm : Gain  Gain=100
  m>mm : Gain  Gain=1000
  mm>  cm : Gain  Gain=.1
  mm>m : Gain  Gain=.001
  psi to Bar : Gain  Gain=.069
  s > min : Gain  Gain=60
  s > min1 : Gain  Gain=60
  PROS1_Permeate : Outport
  PROS1_Brine : Outport  Port=2
  tag scope: PROS1_4_deltaPi=global
  wires:
  Number of Vessels/1 -> Channel Area (m2)/3
  [PROS1_MembraneConstants] -> Bus Selector1/1
  Minus/1 -> Bus Creator1/3  "PROS1_4_ConcentratePressure_psi"
  bar>psi/1 -> Minus/1  "PROS1_4_ConcentratePressure_psi"
  Membrane Width (m)/1 -> Channel Area (m2)/1, m>mm/1
  [RO_PermeatePressure] -> psi to Bar/1  "Permeate Pressure (psi)"
  Spacer Thickness (mm)/1 -> MATLAB Function1/2(h), mm>m/1
  Bus Selector1/3 -> Permeate Flow (gpm)/2  "<PROS1_Area_m2>"
  Inflow/1 -> Bus Selector/1
  Bus Selector1/1 -> initial Units/1  "<PROS1_A>"
  Bus Selector1/2 -> Initial units/1  "<PROS1_B>"
  initial Units/1 -> m3 > L/1
  psi to Bar/1 -> Min/2  "Pressure (bar)"
  Bus Selector/1 -> Min/1, Subsystem/2(<S1 Feed Pressure (bar)>), bar>psi/1  "<S1 Feed Pressure (bar)>"
  Bus Selector/2 -> Brine Flow (gpm)/2, Q (L/min)/1  "<PROS1_4_FeedFlowRate_gpm>"
  Subsystem/2(Permeate Salinity g/L) -> cperm_previous/1, Bus Creator/2, MATLAB Function2/1(cperm)  "PROS1_4_PermeateSalinity_gL"
  Bus Selector/3 -> MATLAB Function2/5(cfeed), Scope1/2, Subsystem/6(<S1 Feed Salinity (g/L)>)  "<S1 Feed Salinity (g/L)>"
  Bus Selector/4 -> Subsystem/1(<Feed Temperature (oC)>)  "<Feed Temperature (oC)>"
  m/min > cm/sec/1 -> Subsystem/11(u)
  Initial units/1 -> m3 > L1/1
  Fouling Factor/1 -> Product2/2
  mm>m/1 -> Channel Area (m2)/2
  Min/1 -> Subsystem/3(Pperm)
  Pa > Bar/1 -> Product2/1  "Water Perm (L/m2/min/Bar)"
  m3 > L/1 -> s > min/1
  Q (L/min)/1 -> Scope1/1, L>m3/1, MATLAB Function2/4(Qfeed)  "Qtot (L/min)"
  "L -> gal"/1 -> Permeate Flow (gpm)/1
  m3 > L1/1 -> s > min1/1
  Elements per Vessel/1 -> Channel Area (m2)/4
  [PROS2_Suction_PressureDrop_psi] -> Minus/2
  s > min/1 -> Pa > Bar/1
  s > min1/1 -> Subsystem/5(Salt Perm (L/m2/min))  "Salt Perm (L/m2/min)"
  m>mm/1 -> MATLAB Function1/1(W)
  MATLAB Function2/1(cbrine) -> Bus Creator1/2  "PROS1_4_BrineConductivity_gL"
  L>m3/1 -> Product/1
  Channel Area (m2)/1 -> Product/2
  cperm_previous/1 -> Subsystem/7(cperm)  "cperm"
  MATLAB Function1/1(dh) -> mm>  cm/1
  Feed Channel Height (m)/1 -> m>cm/1
  Product/1 -> m/min > cm/sec/1
  mm>  cm/1 -> Subsystem/9(dh)
  Product2/1 -> Subsystem/4(Water Perm (L/m2/min/Bar))  "Water Perm (L/m2/min/Bar)"
  m>cm/1 -> Subsystem/10(L)
  Subsystem/1(Permeate Flux Rate (L/min/m2)) -> Jw_Previous/1, "L -> gal"/1  "Permeate Flux Rate* (L/min.m2)"
  Subsystem/3(deltaPi_bar) -> [PROS1_4_deltaPi]
  gpm > L/1 -> MATLAB Function2/3(Qbrine)
  Jw_Previous/1 -> Subsystem/8(Jw)  "Jw"
  Gain/1 -> MATLAB Function2/2(Qperm)  "Predicted Permeate Flow (L/min)"
  Permeate Flow (gpm)/1 -> Brine Flow (gpm)/1, Bus Creator/1, Gain/1  "PROS1_4_PermeateFlow_gpm"
  Bus Creator/1 -> PROS1_Permeate/1  "PRO1_PermeateFlow"
  Brine Flow (gpm)/1 -> Bus Creator1/1, gpm > L/1  "PROS1_4_BrineFlow_gpm"
  Bus Creator1/1 -> PROS1_Brine/1  "PROS1_Feedwater"

== system ARC_DTm/PROS1_4_Pump ==
  note: Determine Needed Added Pressure
  note: gpm / (gpm/psi*ft2) / ft2
  S1 Feed Flow Rate (gpm) : Inport
  Bar > psi : Gain  Gain=1/.069
  Bus Creator : BusCreator  Inputs=4
  Bus Selector : BusSelector  OutputSignals=PROS1_A,PROS1_Area_m2
  Bus Selector1 : BusSelector  OutputSignals=PROS1_4_FeedFlowRate_gpm,PRO_SuctionPressure_psi
  Compare To Constant : simulink/Logic and Bit Operations/Compare To Constant  relop=>  const=1  OutDataTypeStr=boolean
  Constant : Constant  Value=0
  Display{,1..3} (4 alike) : Display
  Gain : Gain  Gain=.01
  Gain3 : Gain  Gain=10.76
  MATLAB Function : MATLAB Function  TreatAsAtomicUnit=on
  Memory : Memory
  PROS1_4_recoveryrate_per : Constant  Value=62
  Pa > psi : Gain  Gain=6895
  Product : Product  Inputs=**/
  Product1 : Product
  Product2 : Product
  Product3 : Product
  Scope : Scope  NumInputPorts=2
      settings: ActiveDisplayYMinimum=-21.182201274193289  ActiveDisplayYMaximum=190.63981146773963  DataLoggingVariableName=ScopeData13
  Scope1 : Scope  NumInputPorts=2
      settings: ActiveDisplayYMinimum=-1  ActiveDisplayYMaximum=1  DataLoggingVariableName=ScopeData14
  Scope3 : Scope
      settings: ActiveDisplayYMinimum=-1  ActiveDisplayYMaximum=1  DataLoggingVariableName=ScopeData16
  Sum : Sum  Inputs=|-+
  Sum1 : Sum  Inputs=|++
  Sum2 : Sum  Inputs=|++
  Switch : Switch  Criteria=u2 > Threshold  SaturateOnIntegerOverflow=off  InputSameDT=off
  m2 > ft2 : Gain  Gain=1/10.76
  m3 > gal : Gain  Gain=264.2
  m3/m2/s/Pa : Gain  Gain=10^-11
  psi to Bar : Gain  Gain=.069
  psi>ft : Gain  Gain=2.31
  s > min : Gain  Gain=60
  PRO1-1 FeedWater Characteristics : Outport
  tag scope: PROS1_4_Power_kW=global
  wires:
  Bus Selector1/2 -> Sum/1  "<PRO_SuctionPressure_psi>"
  Product2/1 -> Bus Creator/1  "S1 Feed Salinity (g/L)"
  [T] -> Bus Creator/2  "Feed Temperature (oC)"
  psi to Bar/1 -> Product3/2  "S1 Feed Pressure (bar)"
  Bus Creator/1 -> PRO1-1 FeedWater Characteristics/1
  [PROS1_4_deltaPi] -> Bar > psi/1
  Switch/1 -> Sum1/2
  Sum1/1 -> Scope3/1, Sum2/1  "Net Opposing Pressure (psi)"
  Bar > psi/1 -> Memory/1
  [PROS1_MembraneConstants] -> Bus Selector/1
  Bus Selector/1 -> m3/m2/s/Pa/1  "<PROS1_A>"
  PROS1_4_recoveryrate_per/1 -> Gain/1
  Gain/1 -> Product/2
  Product/1 -> Sum2/2  "PROS1_4_RequiredNDP_psi"
  m3 > gal/1 -> s > min/1
  s > min/1 -> Pa > psi/1
  m3/m2/s/Pa/1 -> m3 > gal/1
  Pa > psi/1 -> m2 > ft2/1  "Water Perm (gpm/m2/bar)"
  m2 > ft2/1 -> Product1/1  "PROS1_WaterPermeability_gpm_psi_ft2"
  Sum2/1 -> psi to Bar/1, Sum/2, Scope1/1  "PROS1_4_FeedPressure_psi"
  Bus Selector/2 -> Gain3/1  "<PROS1_Area_m2>"
  Gain3/1 -> Display/1, Product1/2  "PROS1_Area_ft2"
  S1 Feed Flow Rate (gpm)/1 -> Bus Selector1/1  "InflowRate (gpm)"
  Sum/1 -> Scope1/2, psi>ft/1
  psi>ft/1 -> Display3/1, MATLAB Function/2(h_des)
  MATLAB Function/2(power) -> [PROS1_4_Power_kW], Scope/1  "PROS1_4_Power_kW"
  Memory/1 -> Sum1/1
  Product1/1 -> Product/3
  MATLAB Function/1(speed) -> Display2/1
  Bus Selector1/1 -> Display1/1, Scope/2, MATLAB Function/1(Q_des), Compare To Constant/1, Bus Creator/3, Switch/2, Product/1  "<PROS1_4_FeedFlowRate_gpm>"
  [PROS1_FeedTDS_gL] -> Product2/1  "S1 Feed Salinity (g/L)"
  Compare To Constant/1 -> Product3/1, Product2/2
  Product3/1 -> Bus Creator/4  "S1 Feed Pressure (bar)"
  [RO_PermeatePressure] -> Switch/1
  Constant/1 -> Switch/3
